simulink model "CVCmodel"  (R2024b)
settings: Solver=VariableStepAuto  StartTime=0.0  StopTime=1  RelTol=0.001
undefined symbols (not defined in the file): Apiston, Arod, d, Dv, E, F, Gint, kd, ki1, kp, Kv, m, omega, Qo, stroke, ymax
settings Model: Creator=ahmed  LastModifiedBy=ahmed
settings DebuggingCC: AlgebraicLoopMsg=none

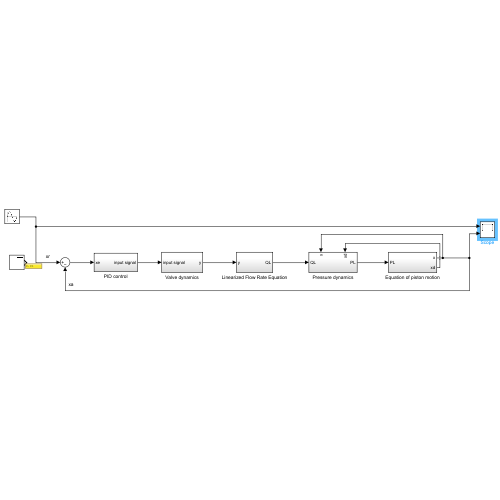
[thumbnail: Simulink's stored preview of the top-level diagram]
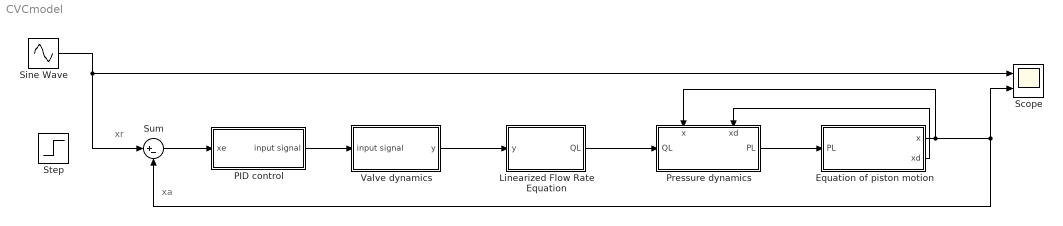
== system CVCmodel ==
  note: xa
  note: xr
  Equation of piston motion : Subsystem
  Linearized Flow Rate Equation : Subsystem
  PID control : Subsystem
  Pressure dynamics : Subsystem
      settings: PortSchema="{\"entries\":[{\"content\":{\"sides\":[{\"content\":{\"connectorIds\":[\"In1\"]},\"type\":\"ConnectorPlacement.EquallySpacedRectSide\",\"uuid\":\"05cf5127-af77-406c-abe5-70f22acd2f7a\"},{\"content\":{\"connectorIds\":[\"Out1\"],\"side\":\"RIGHT\"},\"type\":\"ConnectorPlacement.EquallySpacedRectSide\",\"uuid\":\"84ab6b1f-0882-4366-8b47-aa832abc02c6\"},{\"content\":{\"connectorIds\":[\"In2\",\"In3\"],\"side\":\"TOP\"},\"type\":\"ConnectorPlacement.EquallySpacedRectSide\",\"uuid\":\"4b387211-f687-4226-bfb4-4d710f635374\"},{\"content\":{\"side\":\"BOTTOM\"},\"type\":\"ConnectorPlacement.EquallySpacedRectSide\",\"uuid\":\"d7012891-c30e-43bc-9c6c-d8de03f802fd\"}]},\"type\":\"ConnectorPlacement.EquallySpacedConnector\",\"uuid\":\"a56975bf-2482-4654-8f2c-a1e585f8f660\"}],\"packageUris\":[\"http://schema.mathworks.com/mf0/Connector/R2020b\"],\"version\":\"1.0\"}"
  Scope : Scope  NumInputPorts=2
  Sine Wave : Sin  Amplitude=0.0035  Frequency=31.4  SampleTime=0
  Step : Step  Time=0  After=10e-3  SampleTime=0
  Sum : Sum  Inputs=|+-
  Valve dynamics : Subsystem
  wires:
  Equation of piston motion/1(x) -> Sum/2, Scope/2, Pressure dynamics/2(x)
  Linearized Flow Rate Equation/1(QL) -> Pressure dynamics/1(QL)
  Sum/1 -> PID control/1(xe)
  Valve dynamics/1(y) -> Linearized Flow Rate Equation/1(y)
  PID control/1(input signal) -> Valve dynamics/1(input signal)
  Equation of piston motion/2(xd) -> Pressure dynamics/3(xd)
  Pressure dynamics/1(PL) -> Equation of piston motion/1(PL)
  Sine Wave/1 -> Scope/1, Sum/1

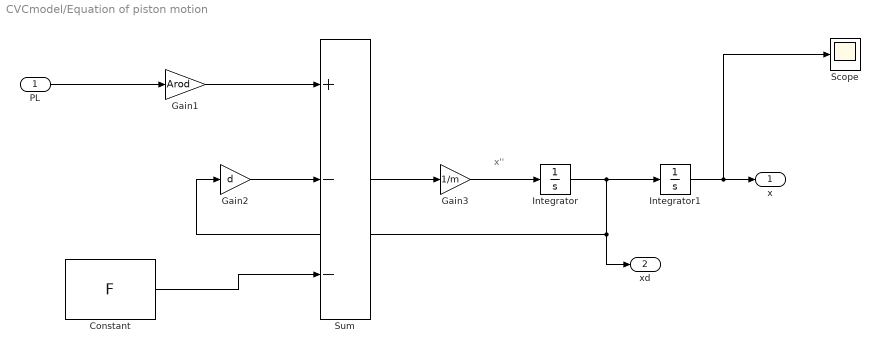
== system CVCmodel/Equation of piston motion ==
  note: x''
  PL : Inport
  Constant : Constant  Value=F
  Gain1 : Gain  Gain=Arod
  Gain2 : Gain  Gain=d
  Gain3 : Gain  Gain=1/m
  Integrator : Integrator
  Integrator1 : Integrator
  Scope : Scope
  Sum : Sum  Inputs=+--
  x : Outport
  xd : Outport  Port=2
  wires:
  Constant/1 -> Sum/3
  Gain2/1 -> Sum/2
  Sum/1 -> Gain3/1
  Gain3/1 -> Integrator/1
  Integrator/1 -> xd/1, Gain2/1, Integrator1/1
  Integrator1/1 -> Scope/1, x/1
  PL/1 -> Gain1/1
  Gain1/1 -> Sum/1

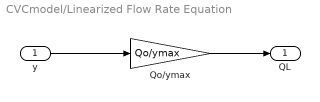
== system CVCmodel/Linearized Flow Rate Equation ==
  y : Inport
  Qo/ymax : Gain  Gain=Qo/ymax
  QL : Outport
  wires:
  y/1 -> Qo/ymax/1
  Qo/ymax/1 -> QL/1

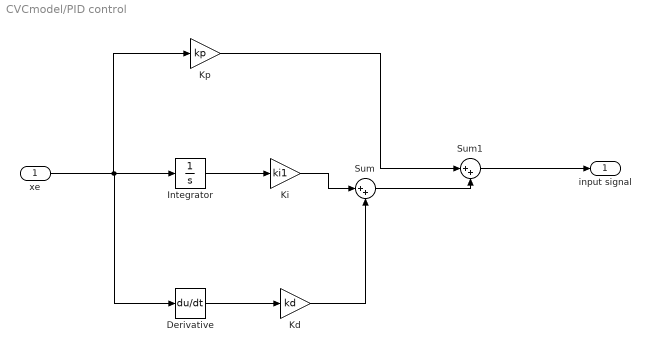
== system CVCmodel/PID control ==
  xe : Inport
  Derivative : Derivative
  Integrator : Integrator
  Kd : Gain  Gain=kd
  Ki : Gain  Gain=ki1
  Kp : Gain  Gain=kp
  Sum : Sum  Inputs=|++
  Sum1 : Sum  Inputs=|++
  input signal : Outport
  wires:
  Sum1/1 -> input signal/1
  xe/1 -> Kp/1, Derivative/1, Integrator/1
  Kp/1 -> Sum1/1
  Integrator/1 -> Ki/1
  Derivative/1 -> Kd/1
  Ki/1 -> Sum/1
  Kd/1 -> Sum/2
  Sum/1 -> Sum1/2

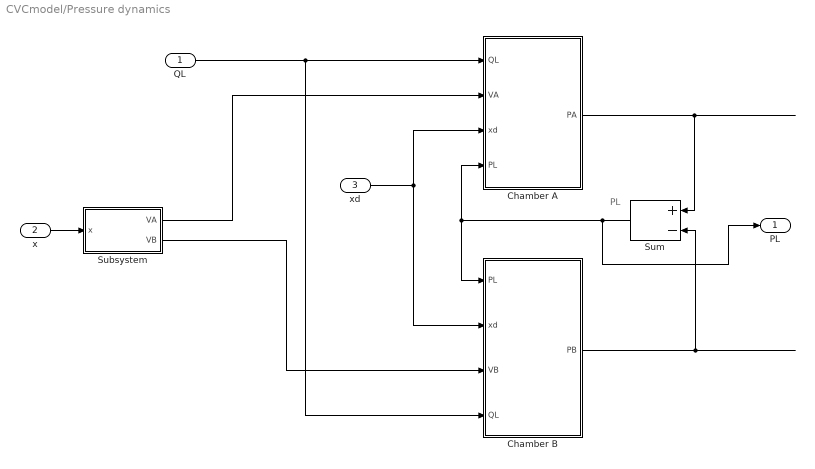
== system CVCmodel/Pressure dynamics ==
  note: PL
  QL : Inport
  x : Inport  Port=2
  xd : Inport  Port=3
  Chamber A : Subsystem
  Chamber B : Subsystem
  Subsystem : Subsystem
  Sum : Sum  Inputs=+|-
  PL : Outport
  wires:
  QL/1 -> Chamber B/4(QL), Chamber A/1(QL)
  xd/1 -> Chamber B/2(xd), Chamber A/3(xd)
  x/1 -> Subsystem/1(x)
  Subsystem/1(VA) -> Chamber A/2(VA)
  Subsystem/2(VB) -> Chamber B/3(VB)
  Chamber B/1(PB) -> Sum/2
  Chamber A/1(PA) -> Sum/1
  Sum/1 -> PL/1, Chamber B/1(PL), Chamber A/4(PL)

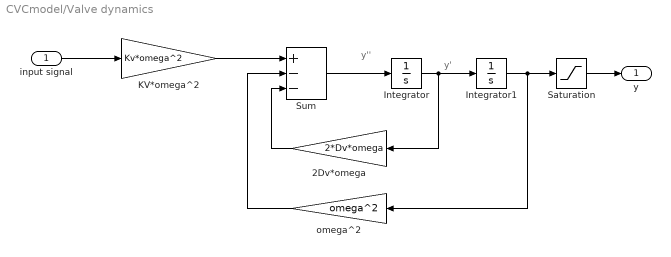
== system CVCmodel/Valve dynamics ==
  note: y'
  note: y''
  input signal : Inport
  2Dv*omega : Gain  Gain=2*Dv*omega
  Integrator : Integrator
  Integrator1 : Integrator
  KV*omega^2 : Gain  Gain=Kv*omega^2
  Saturation : Saturate  UpperLimit=0.001  LowerLimit=-0.001
  Sum : Sum  Inputs=+--
  omega^2 : Gain  Gain=omega^2
  y : Outport
  wires:
  input signal/1 -> KV*omega^2/1
  KV*omega^2/1 -> Sum/1
  Sum/1 -> Integrator/1
  Integrator/1 -> 2Dv*omega/1, Integrator1/1
  Integrator1/1 -> Saturation/1, omega^2/1
  2Dv*omega/1 -> Sum/3
  omega^2/1 -> Sum/2
  Saturation/1 -> y/1

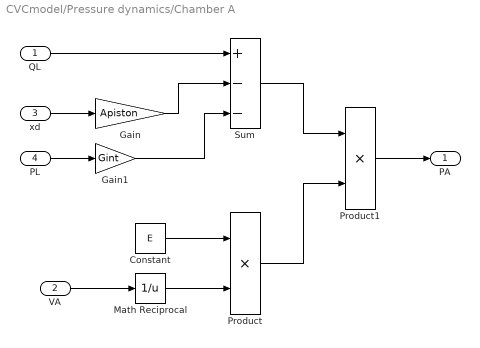
== system CVCmodel/Pressure dynamics/Chamber A ==
  QL : Inport
  VA : Inport  Port=2
  xd : Inport  Port=3
  PL : Inport  Port=4
  Constant : Constant  Value=E
  Gain : Gain  Gain=Apiston
  Gain1 : Gain  Gain=Gint
  Math Reciprocal : Math  Operator=reciprocal  SignedPower=on
  Product : Product
  Product1 : Product
  Sum : Sum  Inputs=+--
  PA : Outport
  wires:
  Constant/1 -> Product/1
  VA/1 -> Math Reciprocal/1
  Math Reciprocal/1 -> Product/2
  QL/1 -> Sum/1
  xd/1 -> Gain/1
  Gain/1 -> Sum/2
  PL/1 -> Gain1/1
  Gain1/1 -> Sum/3
  Sum/1 -> Product1/1
  Product/1 -> Product1/2
  Product1/1 -> PA/1

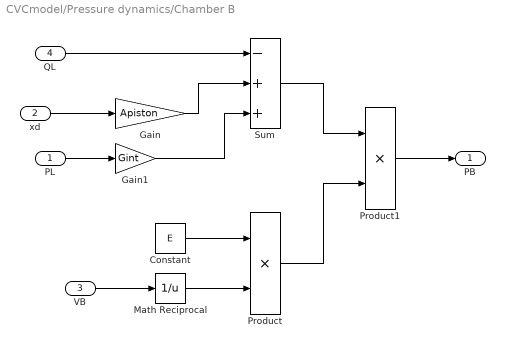
== system CVCmodel/Pressure dynamics/Chamber B ==
  PL : Inport
  xd : Inport  Port=2
  VB : Inport  Port=3
  QL : Inport  Port=4
  Constant : Constant  Value=E
  Gain : Gain  Gain=Apiston
  Gain1 : Gain  Gain=Gint
  Math Reciprocal : Math  Operator=reciprocal  SignedPower=on
  Product : Product
  Product1 : Product
  Sum : Sum  Inputs=-++
  PB : Outport
  wires:
  Gain1/1 -> Sum/3
  QL/1 -> Sum/1
  Sum/1 -> Product1/1
  Product/1 -> Product1/2
  Gain/1 -> Sum/2
  Product1/1 -> PB/1
  VB/1 -> Math Reciprocal/1
  Constant/1 -> Product/1
  Math Reciprocal/1 -> Product/2
  PL/1 -> Gain1/1
  xd/1 -> Gain/1

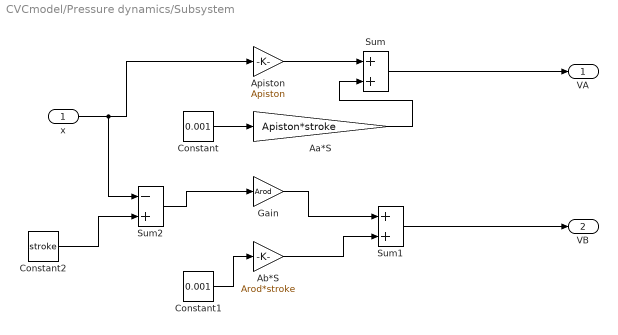
== system CVCmodel/Pressure dynamics/Subsystem ==
  x : Inport
  Aa*S : Gain  Gain=Apiston*stroke
  Ab*S : Gain  Gain=Arod*stroke
  Apiston : Gain  Gain=Apiston
  Constant : Constant  Value=0.001
  Constant1 : Constant  Value=0.001
  Constant2 : Constant  Value=stroke
  Gain : Gain  Gain=Arod
  Sum : Sum
  Sum1 : Sum
  Sum2 : Sum  Inputs=-+
  VA : Outport
  VB : Outport  Port=2
  wires:
  x/1 -> Sum2/1, Apiston/1
  Apiston/1 -> Sum/1
  Sum/1 -> VA/1
  Constant/1 -> Aa*S/1
  Aa*S/1 -> Sum/2
  Sum1/1 -> VB/1
  Constant1/1 -> Ab*S/1
  Ab*S/1 -> Sum1/2
  Constant2/1 -> Sum2/2
  Sum2/1 -> Gain/1
  Gain/1 -> Sum1/1
